simulink model "simpleSum"  (R2019b)
settings: Solver=FixedStepAuto  StartTime=0.0  StopTime=10.0  RelTol=1e-3
model workspace (MAT data in the model file):
  x = Simulink.Parameter
  x.DataType = 'single'
  x.Dimensions = [0 0]
  y = Simulink.Parameter
  y.DataType = 'single'
  y.Dimensions = [0 0]
settings Model: OrderedModelArguments=off  Creator=z003w73w  LastModifiedBy=z003w73w
settings OptimizationCC: OptimizeBlockIOStorage=off  BufferReuse=off  GlobalBufferReuse=off  ExpressionFolding=off  LocalBlockOutputs=off  OptimizeDataStoreBuffers=off  BusAssignmentInplaceUpdate=off
settings DebuggingCC: SFUnexpectedBacktrackingDiag=warning  SFNoUnconditionalDefaultTransitionDiag=warning
settings RTWCC: Description=Create Visual C/C++ Solution File for Simulink Coder  PackageGeneratedCodeAndArtifacts=on  PackageName=simpleSum  TemplateMakefile=RTW.MSVCBuild  GenerateReport=on  BuildConfiguration=Debug  LaunchReport=on
settings CodeAppCC: ForceParamTrailComments=on  MATLABSourceComments=on  EnableCustomComments=on
settings GRTTargetCC: CombineSignalStateStructs=on  MatFileLogging=off  SupportVariableSizeSignals=on  ArrayLayout=Row-major  MultiInstanceErrorCode=Warning

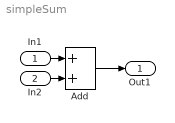
== system simpleSum ==
  In1 : Inport  OutDataTypeStr=single
  In2 : Inport  Port=2  OutDataTypeStr=single
  Add : Sum  AccumDataTypeStr=single  OutDataTypeStr=single
  Out1 : Outport  OutDataTypeStr=single
  wires:
  Add/1 -> Out1/1
  In1/1 -> Add/1
  In2/1 -> Add/2
